simulink library "speedgoatlib_evse"  (R2024b)
settings: Solver=VariableStepAuto  StartTime=0.0  StopTime=10.0  RelTol=1e-3
undefined symbols (not defined in the file): sg_ev_charging_read_m, sg_ev_charging_write_m, sg_ev_isolation_read_m, sg_ev_parameter_read_m, sg_ev_parameter_write_m, sg_ev_precharge_read_m, sg_ev_precharge_write_m, sg_ev_status_m, sg_ev_stop_read_m, sg_ev_stop_write_m, sg_ev_welding_read_m, sg_ev_welding_write_m, sg_evse_charging_read_m, sg_evse_charging_write_m, sg_evse_isolation_read_m, sg_evse_isolation_write_m, sg_evse_parameter_read_m, sg_evse_parameter_write_m, sg_evse_precharge_read_m, sg_evse_precharge_write_m, sg_evse_status_m, sg_evse_stop_read_m, sg_evse_stop_write_m, sg_evse_welding_read_m, sg_evse_welding_write_m
libraries: speedgoatlib_mqtt x199, simulink x39, $bdroot x24
(part 6 of 8)

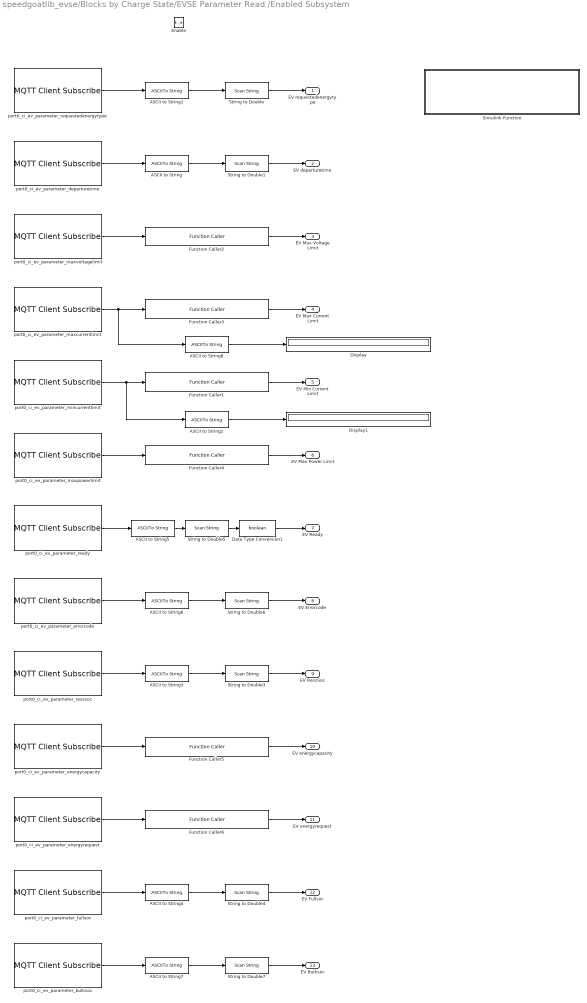
== system speedgoatlib_evse/Blocks by Charge State/EVSE Parameter Read /Enabled Subsystem ==
  Enable : EnablePort
  ASCII to String{,1..8} (9 alike) : ASCIIToString
  Data Type Conversion1 : DataTypeConversion  OutDataTypeStr=boolean  SaturateOnIntegerOverflow=off  RndMeth=Floor
  Display : Display
  Display1 : Display
  Function Caller{1..6} (6 alike) : FunctionCaller  FunctionPrototype=value = fromJsonPhysicalValue(uint8_vec)  InputArgumentSpecifications=zeros(1,48,'uint8')  OutputArgumentSpecifications=double(0)
  Simulink Function : Subsystem  TreatAsAtomicUnit=on
  String to Double{,1,3..7} (7 alike) : ScanString  Format="\"%lf\""
  port0_ci_ev_parameter_bulksoc : speedgoatlib_mqtt/Client/MQTT Client Subscribe  ClientId=parClientId  ConnectionId=parConnectionId  Topic='port0/ci/ev/parameter/bulksoc'  QoS=0 - at most once  InitValue=zeros(1,12,'uint8')  Extended=off  SampleTime=parSampleTime
      settings: SourceProductName=MQTT
  port0_ci_ev_parameter_departuretime : speedgoatlib_mqtt/Client/MQTT Client Subscribe  ClientId=parClientId  ConnectionId=parConnectionId  Topic='port0/ci/ev/parameter/departuretime'  QoS=0 - at most once  InitValue=zeros(1,24,'uint8')  Extended=off  SampleTime=parSampleTime
      settings: SourceProductName=MQTT
  port0_ci_ev_parameter_energycapacity : speedgoatlib_mqtt/Client/MQTT Client Subscribe  ClientId=parClientId  ConnectionId=parConnectionId  Topic='port0/ci/ev/parameter/energycapacity'  QoS=0 - at most once  InitValue=zeros(1,48,'uint8')  Extended=off  SampleTime=parSampleTime
      settings: SourceProductName=MQTT
  port0_ci_ev_parameter_energyrequest : speedgoatlib_mqtt/Client/MQTT Client Subscribe  ClientId=parClientId  ConnectionId=parConnectionId  Topic='port0/ci/ev/parameter/energyrequest'  QoS=0 - at most once  InitValue=zeros(1,48,'uint8')  Extended=off  SampleTime=parSampleTime
      settings: SourceProductName=MQTT
  port0_ci_ev_parameter_errorcode : speedgoatlib_mqtt/Client/MQTT Client Subscribe  ClientId=parClientId  ConnectionId=parConnectionId  Topic='port0/ci/ev/parameter/errorcode'  QoS=0 - at most once  InitValue=zeros(1,24,'uint8')  Extended=off  SampleTime=parSampleTime
      settings: SourceProductName=MQTT
  port0_ci_ev_parameter_fullsoc : speedgoatlib_mqtt/Client/MQTT Client Subscribe  ClientId=parClientId  ConnectionId=parConnectionId  Topic='port0/ci/ev/parameter/fullsoc'  QoS=0 - at most once  InitValue=zeros(1,12,'uint8')  Extended=off  SampleTime=parSampleTime
      settings: SourceProductName=MQTT
  port0_ci_ev_parameter_maxcurrentlimit : speedgoatlib_mqtt/Client/MQTT Client Subscribe  ClientId=parClientId  ConnectionId=parConnectionId  Topic='port0/ci/ev/parameter/maxcurrentlimit'  QoS=0 - at most once  InitValue=zeros(1,48,'uint8')  Extended=off  SampleTime=parSampleTime
      settings: SourceProductName=MQTT
  port0_ci_ev_parameter_maxpowerlimit : speedgoatlib_mqtt/Client/MQTT Client Subscribe  ClientId=parClientId  ConnectionId=parConnectionId  Topic='port0/ci/ev/parameter/maxpowerlimit'  QoS=0 - at most once  InitValue=zeros(1,48,'uint8')  Extended=off  SampleTime=parSampleTime
      settings: SourceProductName=MQTT
  port0_ci_ev_parameter_maxvoltagelimit : speedgoatlib_mqtt/Client/MQTT Client Subscribe  ClientId=parClientId  ConnectionId=parConnectionId  Topic='port0/ci/ev/parameter/maxvoltagelimit'  QoS=0 - at most once  InitValue=zeros(1,48,'uint8')  Extended=off  SampleTime=parSampleTime
      settings: SourceProductName=MQTT
  port0_ci_ev_parameter_mincurrentlimit : speedgoatlib_mqtt/Client/MQTT Client Subscribe  ClientId=parClientId  ConnectionId=parConnectionId  Topic='port0/ci/ev/parameter/mincurrentlimit'  QoS=0 - at most once  InitValue=zeros(1,48,'uint8')  Extended=off  SampleTime=parSampleTime
      settings: SourceProductName=MQTT
  port0_ci_ev_parameter_ready : speedgoatlib_mqtt/Client/MQTT Client Subscribe  ClientId=parClientId  ConnectionId=parConnectionId  Topic='port0/ci/ev/parameter/ready'  QoS=0 - at most once  InitValue=zeros(1,12,'uint8')  Extended=off  SampleTime=parSampleTime
      settings: SourceProductName=MQTT
  port0_ci_ev_parameter_requestedenergytype : speedgoatlib_mqtt/Client/MQTT Client Subscribe  ClientId=parClientId  ConnectionId=parConnectionId  Topic='port0/ci/ev/parameter/requestedenergytype'  QoS=0 - at most once  InitValue=zeros(1,12,'uint8')  Extended=off  SampleTime=parSampleTime
      settings: SourceProductName=MQTT
  port0_ci_ev_parameter_resssoc : speedgoatlib_mqtt/Client/MQTT Client Subscribe  ClientId=parClientId  ConnectionId=parConnectionId  Topic='port0/ci/ev/parameter/resssoc'  QoS=0 - at most once  InitValue=zeros(1,12,'uint8')  Extended=off  SampleTime=parSampleTime
      settings: SourceProductName=MQTT
  EV requestedenergytype : Outport
  EV departuretime : Outport  Port=2
  EV Max Voltage Limit : Outport  Port=3
  EV Max Current Limit : Outport  Port=4
  EV Min Current Limit : Outport  Port=5
  EV Max Power Limit : Outport  Port=6
  EV Ready : Outport  Port=7
  EV Errorcode : Outport  Port=8
  EV RessSoc : Outport  Port=9
  EV energycapacity : Outport  Port=10
  EV energyrequest : Outport  Port=11
  EV Fullsoc : Outport  Port=12
  EV Bulksoc : Outport  Port=13
  wires:
  String to Double/1 -> EV requestedenergytype/1
  port0_ci_ev_parameter_maxpowerlimit/1 -> Function Caller4/1
  Function Caller4/1 -> EV Max Power Limit/1
  Function Caller3/1 -> EV Max Current Limit/1
  port0_ci_ev_parameter_maxvoltagelimit/1 -> Function Caller2/1
  Function Caller2/1 -> EV Max Voltage Limit/1
  String to Double1/1 -> EV departuretime/1
  ASCII to String1/1 -> String to Double/1
  ASCII to String/1 -> String to Double1/1
  port0_ci_ev_parameter_departuretime/1 -> ASCII to String/1
  port0_ci_ev_parameter_requestedenergytype/1 -> ASCII to String1/1
  port0_ci_ev_parameter_mincurrentlimit/1 -> ASCII to String2/1, Function Caller1/1
  Function Caller1/1 -> EV Min Current Limit/1
  Data Type Conversion1/1 -> EV Ready/1
  String to Double5/1 -> Data Type Conversion1/1
  ASCII to String5/1 -> String to Double5/1
  port0_ci_ev_parameter_ready/1 -> ASCII to String5/1
  String to Double6/1 -> EV Errorcode/1
  ASCII to String6/1 -> String to Double6/1
  port0_ci_ev_parameter_errorcode/1 -> ASCII to String6/1
  port0_ci_ev_parameter_resssoc/1 -> ASCII to String3/1
  ASCII to String3/1 -> String to Double3/1
  String to Double3/1 -> EV RessSoc/1
  Function Caller5/1 -> EV energycapacity/1
  port0_ci_ev_parameter_energycapacity/1 -> Function Caller5/1
  port0_ci_ev_parameter_energyrequest/1 -> Function Caller6/1
  Function Caller6/1 -> EV energyrequest/1
  String to Double4/1 -> EV Fullsoc/1
  ASCII to String4/1 -> String to Double4/1
  port0_ci_ev_parameter_fullsoc/1 -> ASCII to String4/1
  port0_ci_ev_parameter_bulksoc/1 -> ASCII to String7/1
  ASCII to String7/1 -> String to Double7/1
  String to Double7/1 -> EV Bulksoc/1
  port0_ci_ev_parameter_maxcurrentlimit/1 -> ASCII to String8/1, Function Caller3/1
  ASCII to String8/1 -> Display/1
  ASCII to String2/1 -> Display1/1

== system speedgoatlib_evse/Blocks by Charge State/EVSE Parameter Read /string compare logic ==
  Input : Inport
  ASCII to String1 : ASCIIToString
  Add : Sum
  Data Type Conversion : DataTypeConversion  OutDataTypeStr=double  SaturateOnIntegerOverflow=off  RndMeth=Floor
  Data Type Conversion1 : DataTypeConversion  OutDataTypeStr=double  SaturateOnIntegerOverflow=off  RndMeth=Floor
  Gain : Gain  Gain=2
  String Compare : StringCompare
  String Compare1 : StringCompare
  String Constant : StringConstant  String="\"started\""
  String Constant1 : StringConstant  String="\"finished\""
  Out1 : Outport
  wires:
  ASCII to String1/1 -> String Compare1/1, String Compare/1
  String Constant1/1 -> String Compare1/2
  String Compare/1 -> Data Type Conversion/1
  String Constant/1 -> String Compare/2
  String Compare1/1 -> Data Type Conversion1/1
  Gain/1 -> Add/2
  Add/1 -> Out1/1
  Input/1 -> ASCII to String1/1
  Data Type Conversion/1 -> Add/1
  Data Type Conversion1/1 -> Gain/1

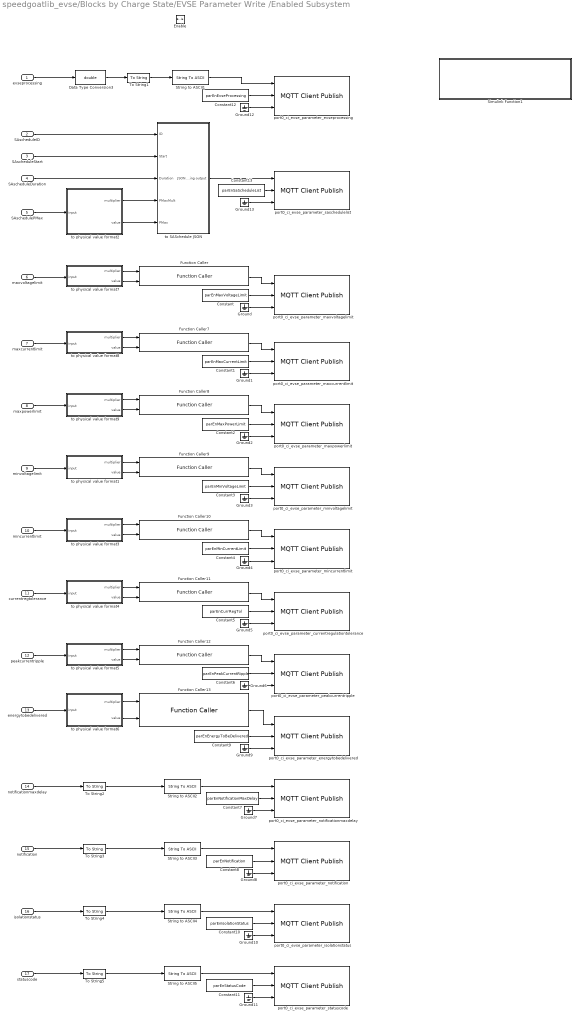
== system speedgoatlib_evse/Blocks by Charge State/EVSE Parameter Write /Enabled Subsystem ==
  evseprocessing : Inport
  SAscheduleID : Inport  Port=2
  SAscheduleStart : Inport  Port=3
  SAscheduleDuration : Inport  Port=4
  SAschedulePMax : Inport  Port=5
  maxvoltagelimit : Inport  Port=6
  maxcurrentlimit : Inport  Port=7
  maxpowerlimit : Inport  Port=8
  minvoltagelimit : Inport  Port=9
  mincurrentlimit : Inport  Port=10
  currentregtolerance : Inport  Port=11
  peakcurrentripple : Inport  Port=12
  energytobedelivered : Inport  Port=13
  notificationmaxdelay : Inport  Port=14
  notification : Inport  Port=15
  isolationstatus : Inport  Port=16
  statuscode : Inport  Port=17
  Enable : EnablePort
  Constant : Constant  Value=parEnMaxVoltageLimit  OutDataTypeStr=boolean
  Constant1 : Constant  Value=parEnMaxCurrentLimit  OutDataTypeStr=boolean
  Constant10 : Constant  Value=parEnIsolationStatus  OutDataTypeStr=boolean
  Constant11 : Constant  Value=parEnStatusCode  OutDataTypeStr=boolean
  Constant12 : Constant  Value=parEnEvseProcessing  OutDataTypeStr=boolean
  Constant13 : Constant  Value=parEnSaScheduleList  OutDataTypeStr=boolean
  Constant2 : Constant  Value=parEnMaxPowerLimit  OutDataTypeStr=boolean
  Constant3 : Constant  Value=parEnMinVoltageLimit  OutDataTypeStr=boolean
  Constant4 : Constant  Value=parEnMinCurrentLimit  OutDataTypeStr=boolean
  Constant5 : Constant  Value=parEnCurrRegTol  OutDataTypeStr=boolean
  Constant6 : Constant  Value=parEnPeakCurrentRipple  OutDataTypeStr=boolean
  Constant7 : Constant  Value=parEnNotificationMaxDelay  OutDataTypeStr=boolean
  Constant8 : Constant  Value=parEnNotification  OutDataTypeStr=boolean
  Constant9 : Constant  Value=parEnEnergyToBeDelivered  OutDataTypeStr=boolean
  Data Type Conversion3 : DataTypeConversion  OutDataTypeStr=double  SaturateOnIntegerOverflow=off  RndMeth=Floor
  Function Caller{,7..13} (8 alike) : FunctionCaller  FunctionPrototype=json_string = toJsonPhysicalValue(multiplier,value)  InputArgumentSpecifications=double(0), double(0)  OutputArgumentSpecifications=zeros(1,48,'uint8')
  Ground{,1..13} (14 alike) : Ground
  Simulink Function1 : Subsystem  TreatAsAtomicUnit=on
  String to ASCII1 : StringToASCII  OutputVectorSize=12
  String to ASCII2 : StringToASCII  OutputVectorSize=16
  String to ASCII3 : StringToASCII  OutputVectorSize=16
  String to ASCII4 : StringToASCII  OutputVectorSize=12
  String to ASCII5 : StringToASCII  OutputVectorSize=12
  To String{1..5} (5 alike) : ToString
  port0_ci_evse_parameter_currentregulationtolerance : speedgoatlib_mqtt/Client/MQTT Client Publish  ClientId=parClientId  ConnectionId=parConnectionId  Topic='port0/ci/evse/parameter/currentregulationtolerance'  QoS=0 - at most once  Retain=on  Extended=on  SampleTime=parSampleTime
      settings: SourceProductName=MQTT
  port0_ci_evse_parameter_energytobedelivered : speedgoatlib_mqtt/Client/MQTT Client Publish  ClientId=parClientId  ConnectionId=parConnectionId  Topic='port0/ci/evse/parameter/energytobedelivered'  QoS=0 - at most once  Retain=on  Extended=on  SampleTime=parSampleTime
      settings: SourceProductName=MQTT
  port0_ci_evse_parameter_evseprocessing : speedgoatlib_mqtt/Client/MQTT Client Publish  ClientId=parClientId  ConnectionId=parConnectionId  Topic='port0/ci/evse/parameter/evseprocessing'  QoS=0 - at most once  Retain=on  Extended=on  SampleTime=parSampleTime
      settings: SourceProductName=MQTT
  port0_ci_evse_parameter_isolationstatus : speedgoatlib_mqtt/Client/MQTT Client Publish  ClientId=parClientId  ConnectionId=parConnectionId  Topic='port0/ci/evse/parameter/isolationstatus'  QoS=0 - at most once  Retain=on  Extended=on  SampleTime=parSampleTime
      settings: SourceProductName=MQTT
  port0_ci_evse_parameter_maxcurrentlimit : speedgoatlib_mqtt/Client/MQTT Client Publish  ClientId=parClientId  ConnectionId=parConnectionId  Topic='port0/ci/evse/parameter/maxcurrentlimit'  QoS=0 - at most once  Retain=on  Extended=on  SampleTime=parSampleTime
      settings: SourceProductName=MQTT
  port0_ci_evse_parameter_maxpowerlimit : speedgoatlib_mqtt/Client/MQTT Client Publish  ClientId=parClientId  ConnectionId=parConnectionId  Topic='port0/ci/evse/parameter/maxpowerlimit'  QoS=0 - at most once  Retain=on  Extended=on  SampleTime=parSampleTime
      settings: SourceProductName=MQTT
  port0_ci_evse_parameter_maxvoltagelimit : speedgoatlib_mqtt/Client/MQTT Client Publish  ClientId=parClientId  ConnectionId=parConnectionId  Topic='port0/ci/evse/parameter/maxvoltagelimit'  QoS=0 - at most once  Retain=on  Extended=on  SampleTime=parSampleTime
      settings: SourceProductName=MQTT
  port0_ci_evse_parameter_mincurrentlimit : speedgoatlib_mqtt/Client/MQTT Client Publish  ClientId=parClientId  ConnectionId=parConnectionId  Topic='port0/ci/evse/parameter/mincurrentlimit'  QoS=0 - at most once  Retain=on  Extended=on  SampleTime=parSampleTime
      settings: SourceProductName=MQTT
  port0_ci_evse_parameter_minvoltagelimit : speedgoatlib_mqtt/Client/MQTT Client Publish  ClientId=parClientId  ConnectionId=parConnectionId  Topic='port0/ci/evse/parameter/minvoltagelimit'  QoS=0 - at most once  Retain=on  Extended=on  SampleTime=parSampleTime
      settings: SourceProductName=MQTT
  port0_ci_evse_parameter_notification : speedgoatlib_mqtt/Client/MQTT Client Publish  ClientId=parClientId  ConnectionId=parConnectionId  Topic='port0/ci/evse/parameter/notification'  QoS=0 - at most once  Retain=on  Extended=on  SampleTime=parSampleTime
      settings: SourceProductName=MQTT
  port0_ci_evse_parameter_notificationmaxdelay : speedgoatlib_mqtt/Client/MQTT Client Publish  ClientId=parClientId  ConnectionId=parConnectionId  Topic='port0/ci/evse/parameter/notificationmaxdelay'  QoS=0 - at most once  Retain=on  Extended=on  SampleTime=parSampleTime
      settings: SourceProductName=MQTT
  port0_ci_evse_parameter_peakcurrentripple : speedgoatlib_mqtt/Client/MQTT Client Publish  ClientId=parClientId  ConnectionId=parConnectionId  Topic='port0/ci/evse/parameter/peakcurrentripple'  QoS=0 - at most once  Retain=on  Extended=on  SampleTime=parSampleTime
      settings: SourceProductName=MQTT
  port0_ci_evse_parameter_saschedulelist : speedgoatlib_mqtt/Client/MQTT Client Publish  ClientId=parClientId  ConnectionId=parConnectionId  Topic='port0/ci/evse/parameter/saschedulelist'  QoS=0 - at most once  Retain=on  Extended=on  SampleTime=parSampleTime
      settings: SourceProductName=MQTT
  port0_ci_evse_parameter_statuscode : speedgoatlib_mqtt/Client/MQTT Client Publish  ClientId=parClientId  ConnectionId=parConnectionId  Topic='port0/ci/evse/parameter/statuscode'  QoS=0 - at most once  Retain=on  Extended=on  SampleTime=parSampleTime
      settings: SourceProductName=MQTT
  to SASchedule JSON : Subsystem
  to physical value format1 : MATLAB Function  TreatAsAtomicUnit=on
  to physical value format2 : MATLAB Function  TreatAsAtomicUnit=on
  to physical value format3 : MATLAB Function  TreatAsAtomicUnit=on
  to physical value format4 : MATLAB Function  TreatAsAtomicUnit=on
  to physical value format5 : MATLAB Function  TreatAsAtomicUnit=on
  to physical value format6 : MATLAB Function  TreatAsAtomicUnit=on
  to physical value format7 : MATLAB Function  TreatAsAtomicUnit=on
  to physical value format8 : MATLAB Function  TreatAsAtomicUnit=on
  to physical value format9 : MATLAB Function  TreatAsAtomicUnit=on
  wires:
  to physical value format6/2(value) -> Function Caller13/2
  to physical value format6/1(multiplier) -> Function Caller13/1
  Function Caller13/1 -> port0_ci_evse_parameter_energytobedelivered/1
  Function Caller12/1 -> port0_ci_evse_parameter_peakcurrentripple/1
  to physical value format5/2(value) -> Function Caller12/2
  to physical value format5/1(multiplier) -> Function Caller12/1
  Function Caller11/1 -> port0_ci_evse_parameter_currentregulationtolerance/1
  to physical value format4/2(value) -> Function Caller11/2
  to physical value format4/1(multiplier) -> Function Caller11/1
  Function Caller10/1 -> port0_ci_evse_parameter_mincurrentlimit/1
  to physical value format3/2(value) -> Function Caller10/2
  to physical value format3/1(multiplier) -> Function Caller10/1
  Function Caller9/1 -> port0_ci_evse_parameter_minvoltagelimit/1
  to physical value format1/2(value) -> Function Caller9/2
  to physical value format1/1(multiplier) -> Function Caller9/1
  Function Caller8/1 -> port0_ci_evse_parameter_maxpowerlimit/1
  to physical value format9/2(value) -> Function Caller8/2
  to physical value format9/1(multiplier) -> Function Caller8/1
  Function Caller7/1 -> port0_ci_evse_parameter_maxcurrentlimit/1
  to physical value format8/2(value) -> Function Caller7/2
  to physical value format8/1(multiplier) -> Function Caller7/1
  to physical value format7/2(value) -> Function Caller/2
  to physical value format7/1(multiplier) -> Function Caller/1
  Function Caller/1 -> port0_ci_evse_parameter_maxvoltagelimit/1
  Ground8/1 -> port0_ci_evse_parameter_notification/3
  Constant8/1 -> port0_ci_evse_parameter_notification/2
  Constant7/1 -> port0_ci_evse_parameter_notificationmaxdelay/2
  Ground7/1 -> port0_ci_evse_parameter_notificationmaxdelay/3
  Ground6/1 -> port0_ci_evse_parameter_peakcurrentripple/3
  Constant6/1 -> port0_ci_evse_parameter_peakcurrentripple/2
  Ground5/1 -> port0_ci_evse_parameter_currentregulationtolerance/3
  Constant5/1 -> port0_ci_evse_parameter_currentregulationtolerance/2
  Constant4/1 -> port0_ci_evse_parameter_mincurrentlimit/2
  Ground4/1 -> port0_ci_evse_parameter_mincurrentlimit/3
  Ground3/1 -> port0_ci_evse_parameter_minvoltagelimit/3
  Constant3/1 -> port0_ci_evse_parameter_minvoltagelimit/2
  Constant2/1 -> port0_ci_evse_parameter_maxpowerlimit/2
  Ground2/1 -> port0_ci_evse_parameter_maxpowerlimit/3
  Ground1/1 -> port0_ci_evse_parameter_maxcurrentlimit/3
  Constant1/1 -> port0_ci_evse_parameter_maxcurrentlimit/2
  Constant/1 -> port0_ci_evse_parameter_maxvoltagelimit/2
  Ground/1 -> port0_ci_evse_parameter_maxvoltagelimit/3
  evseprocessing/1 -> Data Type Conversion3/1
  statuscode/1 -> To String5/1
  String to ASCII5/1 -> port0_ci_evse_parameter_statuscode/1
  To String5/1 -> String to ASCII5/1
  To String4/1 -> String to ASCII4/1
  String to ASCII4/1 -> port0_ci_evse_parameter_isolationstatus/1
  isolationstatus/1 -> To String4/1
  notification/1 -> To String3/1
  String to ASCII3/1 -> port0_ci_evse_parameter_notification/1
  To String3/1 -> String to ASCII3/1
  To String2/1 -> String to ASCII2/1
  String to ASCII2/1 -> port0_ci_evse_parameter_notificationmaxdelay/1
  notificationmaxdelay/1 -> To String2/1
  energytobedelivered/1 -> to physical value format6/1(input)
  peakcurrentripple/1 -> to physical value format5/1(input)
  currentregtolerance/1 -> to physical value format4/1(input)
  minvoltagelimit/1 -> to physical value format1/1(input)
  mincurrentlimit/1 -> to physical value format3/1(input)
  to physical value format2/2(value) -> to SASchedule JSON/5(PMax)
  to physical value format2/1(multiplier) -> to SASchedule JSON/4(PMaxMult)
  SAscheduleDuration/1 -> to SASchedule JSON/3(Duration)
  SAscheduleStart/1 -> to SASchedule JSON/2(Start)
  SAscheduleID/1 -> to SASchedule JSON/1(ID)
  SAschedulePMax/1 -> to physical value format2/1(input)
  maxpowerlimit/1 -> to physical value format9/1(input)
  maxcurrentlimit/1 -> to physical value format8/1(input)
  maxvoltagelimit/1 -> to physical value format7/1(input)
  String to ASCII1/1 -> port0_ci_evse_parameter_evseprocessing/1
  to SASchedule JSON/1(JSON string output) -> port0_ci_evse_parameter_saschedulelist/1
  Data Type Conversion3/1 -> To String1/1
  To String1/1 -> String to ASCII1/1
  Constant9/1 -> port0_ci_evse_parameter_energytobedelivered/2
  Ground9/1 -> port0_ci_evse_parameter_energytobedelivered/3
  Constant10/1 -> port0_ci_evse_parameter_isolationstatus/2
  Ground10/1 -> port0_ci_evse_parameter_isolationstatus/3
  Ground11/1 -> port0_ci_evse_parameter_statuscode/3
  Constant11/1 -> port0_ci_evse_parameter_statuscode/2
  Ground12/1 -> port0_ci_evse_parameter_evseprocessing/3
  Constant12/1 -> port0_ci_evse_parameter_evseprocessing/2
  Constant13/1 -> port0_ci_evse_parameter_saschedulelist/2
  Ground13/1 -> port0_ci_evse_parameter_saschedulelist/3

== system speedgoatlib_evse/Blocks by Charge State/EVSE Parameter Write /string compare logic ==
  Input : Inport
  ASCII to String1 : ASCIIToString
  Add : Sum
  Data Type Conversion : DataTypeConversion  OutDataTypeStr=double  SaturateOnIntegerOverflow=off  RndMeth=Floor
  Data Type Conversion1 : DataTypeConversion  OutDataTypeStr=double  SaturateOnIntegerOverflow=off  RndMeth=Floor
  Gain : Gain  Gain=2
  String Compare : StringCompare
  String Compare1 : StringCompare
  String Constant : StringConstant  String="\"started\""
  String Constant1 : StringConstant  String="\"finished\""
  Out1 : Outport
  wires:
  Input/1 -> ASCII to String1/1
  Add/1 -> Out1/1
  Gain/1 -> Add/2
  String Compare1/1 -> Data Type Conversion1/1
  String Constant/1 -> String Compare/2
  String Compare/1 -> Data Type Conversion/1
  String Constant1/1 -> String Compare1/2
  ASCII to String1/1 -> String Compare/1, String Compare1/1
  Data Type Conversion/1 -> Add/1
  Data Type Conversion1/1 -> Gain/1

== system speedgoatlib_evse/Blocks by Charge State/EVSE Pre-Charge Read /Enabled Subsystem ==
  Enable : EnablePort
  ASCII to String : ASCIIToString
  ASCII to String1 : ASCIIToString
  ASCII to String2 : ASCIIToString
  Data Type Conversion1 : DataTypeConversion  OutDataTypeStr=boolean  SaturateOnIntegerOverflow=off  RndMeth=Floor
  Function Caller : FunctionCaller  FunctionPrototype=value = fromJsonPhysicalValue(uint8_vec)  InputArgumentSpecifications=zeros(1,48,'uint8')  OutputArgumentSpecifications=double(0)
  Function Caller1 : FunctionCaller  FunctionPrototype=value = fromJsonPhysicalValue(uint8_vec)  InputArgumentSpecifications=zeros(1,48,'uint8')  OutputArgumentSpecifications=double(0)
  Simulink Function : Subsystem  TreatAsAtomicUnit=on
  String to Double : ScanString  Format="\"%lf\""
  String to Double1 : ScanString  Format="\"%lf\""
  String to Double2 : ScanString  Format="\"%lf\""
  port0_ci_ev_precharge_errorcode : S-Function  FunctionName=sg_mqtt_client_subscribe_s  Parameters="ClientId,  ConnectionId, Topic, QoS, InitValue, Extended, SampleTime"  SFunctionDeploymentMode=off  EnableBusSupport=off  mask(mqtt_client_subscribe_1){ClientId=parClientId, ConnectionId=parConnectionId, Topic='port0/ci/ev/precharge/errorcode', QoS=0 - at most once, InitValue=zeros(1,24,'uint8'), Extended=off, SampleTime=parSampleTime}
      mask prompts: ClientId "Station ID"; ConnectionId "Connection ID"; QoS "Quality of Service"; InitValue "Init Value"; Extended "Extended Interface"; SampleTime "Sample Time [s]"
      mask help: Speedgoat Driver Block<br>MQTT Client - Subscribe<br><br>&copy; 2007 - 2023, Speedgoat GmbH, <a href="matlab: web('www.speedgoat.com','-browser');">www.speedgoat.com</a>
      mask init:
      | sg_mqtt_client_subscribe_m.runMaskInitialization(ClientId, ConnectionId, Topic, InitValue, Extended);
      mask Help: eval('sg.utils.help.show(''io_main/refentry_mqtt_client_subscribe'');')
      mask TypeOptions QoS: 0 - at most once | 1 - at least once | 2 - exactly once
      mask DialogControl groupParameters Prompt: Parameters
      mask Display: disp('Speedgoat\nMQTT Client\nSubscribe\nStation ID: 0\nConnection ID: 0');
  port0_ci_ev_precharge_ready : speedgoatlib_mqtt/Client/MQTT Client Subscribe  ClientId=parClientId  ConnectionId=parConnectionId  Topic='port0/ci/ev/precharge/ready'  QoS=0 - at most once  InitValue=zeros(1,12,'uint8')  Extended=off  SampleTime=parSampleTime
      settings: SourceProductName=MQTT
  port0_ci_ev_precharge_resssoc : S-Function  FunctionName=sg_mqtt_client_subscribe_s  Parameters="ClientId,  ConnectionId, Topic, QoS, InitValue, Extended, SampleTime"  SFunctionDeploymentMode=off  EnableBusSupport=off  mask(mqtt_client_subscribe_1){ClientId=parClientId, ConnectionId=parConnectionId, Topic='port0/ci/ev/precharge/resssoc', QoS=0 - at most once, InitValue=zeros(1,24,'uint8'), Extended=off, SampleTime=parSampleTime}
      mask prompts: ClientId "Station ID"; ConnectionId "Connection ID"; QoS "Quality of Service"; InitValue "Init Value"; Extended "Extended Interface"; SampleTime "Sample Time [s]"
      mask help: Speedgoat Driver Block<br>MQTT Client - Subscribe<br><br>&copy; 2007 - 2023, Speedgoat GmbH, <a href="matlab: web('www.speedgoat.com','-browser');">www.speedgoat.com</a>
      mask init:
      | sg_mqtt_client_subscribe_m.runMaskInitialization(ClientId, ConnectionId, Topic, InitValue, Extended);
      mask Help: eval('sg.utils.help.show(''io_main/refentry_mqtt_client_subscribe'');')
      mask TypeOptions QoS: 0 - at most once | 1 - at least once | 2 - exactly once
      mask DialogControl groupParameters Prompt: Parameters
      mask Display: disp('Speedgoat\nMQTT Client\nSubscribe\nStation ID: 0\nConnection ID: 0');
  port0_ci_ev_precharge_targetcurrent : S-Function  FunctionName=sg_mqtt_client_subscribe_s  Parameters="ClientId,  ConnectionId, Topic, QoS, InitValue, Extended, SampleTime"  SFunctionDeploymentMode=off  EnableBusSupport=off  mask(mqtt_client_subscribe_1){ClientId=parClientId, ConnectionId=parConnectionId, Topic='port0/ci/ev/precharge/targetcurrent', QoS=0 - at most once, InitValue=zeros(1,48,'uint8'), Extended=off, SampleTime=parSampleTime}
      mask prompts: ClientId "Station ID"; ConnectionId "Connection ID"; QoS "Quality of Service"; InitValue "Init Value"; Extended "Extended Interface"; SampleTime "Sample Time [s]"
      mask help: Speedgoat Driver Block<br>MQTT Client - Subscribe<br><br>&copy; 2007 - 2023, Speedgoat GmbH, <a href="matlab: web('www.speedgoat.com','-browser');">www.speedgoat.com</a>
      mask init:
      | sg_mqtt_client_subscribe_m.runMaskInitialization(ClientId, ConnectionId, Topic, InitValue, Extended);
      mask Help: eval('sg.utils.help.show(''io_main/refentry_mqtt_client_subscribe'');')
      mask TypeOptions QoS: 0 - at most once | 1 - at least once | 2 - exactly once
      mask DialogControl groupParameters Prompt: Parameters
      mask Display: disp('Speedgoat\nMQTT Client\nSubscribe\nStation ID: 0\nConnection ID: 0');
  port0_ci_ev_precharge_targetvoltage : S-Function  FunctionName=sg_mqtt_client_subscribe_s  Parameters="ClientId,  ConnectionId, Topic, QoS, InitValue, Extended, SampleTime"  SFunctionDeploymentMode=off  EnableBusSupport=off  mask(mqtt_client_subscribe_1){ClientId=parClientId, ConnectionId=parConnectionId, Topic='port0/ci/ev/precharge/targetvoltage', QoS=0 - at most once, InitValue=zeros(1,48,'uint8'), Extended=off, SampleTime=parSampleTime}
      mask prompts: ClientId "Station ID"; ConnectionId "Connection ID"; QoS "Quality of Service"; InitValue "Init Value"; Extended "Extended Interface"; SampleTime "Sample Time [s]"
      mask help: Speedgoat Driver Block<br>MQTT Client - Subscribe<br><br>&copy; 2007 - 2023, Speedgoat GmbH, <a href="matlab: web('www.speedgoat.com','-browser');">www.speedgoat.com</a>
      mask init:
      | sg_mqtt_client_subscribe_m.runMaskInitialization(ClientId, ConnectionId, Topic, InitValue, Extended);
      mask Help: eval('sg.utils.help.show(''io_main/refentry_mqtt_client_subscribe'');')
      mask TypeOptions QoS: 0 - at most once | 1 - at least once | 2 - exactly once
      mask DialogControl groupParameters Prompt: Parameters
      mask Display: disp('Speedgoat\nMQTT Client\nSubscribe\nStation ID: 0\nConnection ID: 0');
  EV Ready : Outport
  EV Errorcode : Outport  Port=2
  EV RESS SOC : Outport  Port=3
  EV Target Voltage : Outport  Port=4
  EV Target Current : Outport  Port=5
  wires:
  port0_ci_ev_precharge_ready/1 -> ASCII to String1/1
  port0_ci_ev_precharge_errorcode/1 -> ASCII to String/1
  ASCII to String/1 -> String to Double1/1
  ASCII to String1/1 -> String to Double/1
  String to Double/1 -> Data Type Conversion1/1
  String to Double1/1 -> EV Errorcode/1
  String to Double2/1 -> EV RESS SOC/1
  ASCII to String2/1 -> String to Double2/1
  port0_ci_ev_precharge_resssoc/1 -> ASCII to String2/1
  Function Caller/1 -> EV Target Voltage/1
  port0_ci_ev_precharge_targetvoltage/1 -> Function Caller/1
  port0_ci_ev_precharge_targetcurrent/1 -> Function Caller1/1
  Function Caller1/1 -> EV Target Current/1
  Data Type Conversion1/1 -> EV Ready/1

== system speedgoatlib_evse/Blocks by Charge State/EVSE Pre-Charge Read /string compare logic ==
  Input : Inport
  ASCII to String1 : ASCIIToString
  Add : Sum
  Gain : Gain  Gain=2
  String Compare : StringCompare
  String Compare1 : StringCompare
  String Constant : StringConstant  String="\"started\""
  String Constant1 : StringConstant  String="\"finished\""
  Out1 : Outport
  wires:
  Input/1 -> ASCII to String1/1
  Add/1 -> Out1/1
  Gain/1 -> Add/2
  String Compare1/1 -> Gain/1
  String Constant/1 -> String Compare/2
  String Compare/1 -> Add/1
  String Constant1/1 -> String Compare1/2
  ASCII to String1/1 -> String Compare/1, String Compare1/1

== system speedgoatlib_evse/Blocks by Charge State/EVSE Pre-Charge Write /Enabled Subsystem ==
  isolationstatus : Inport
  statuscode : Inport  Port=2
  presentvoltage : Inport  Port=3
  Enable : EnablePort
  Constant : Constant  Value=parEnIsolationStatus  OutDataTypeStr=boolean
  Constant1 : Constant  Value=parEnStatusCode  OutDataTypeStr=boolean
  Constant2 : Constant  Value=parEnPresentVoltage  OutDataTypeStr=boolean
  Data Type Conversion3 : DataTypeConversion  OutDataTypeStr=double  SaturateOnIntegerOverflow=off  RndMeth=Floor
  Data Type Conversion4 : DataTypeConversion  OutDataTypeStr=double  SaturateOnIntegerOverflow=off  RndMeth=Floor
  Function Caller11 : FunctionCaller  FunctionPrototype=json_string = toJsonPhysicalValue(multiplier,value)  InputArgumentSpecifications=double(0), double(0)  OutputArgumentSpecifications=zeros(1,48,'uint8')
  Ground : Ground
  Ground1 : Ground
  Ground2 : Ground
  Simulink Function2 : Subsystem  TreatAsAtomicUnit=on
  String to ASCII1 : StringToASCII  OutputVectorSize=12
  String to ASCII2 : StringToASCII  OutputVectorSize=12
  To String1 : ToString
  To String2 : ToString
  port0_ci_evse_precharge_isolationstatus : speedgoatlib_mqtt/Client/MQTT Client Publish  ClientId=parClientId  ConnectionId=parConnectionId  Topic='port0/ci/evse/precharge/isolationstatus'  QoS=0 - at most once  Retain=on  Extended=on  SampleTime=parSampleTime
      settings: SourceProductName=MQTT
  port0_ci_evse_precharge_presentvoltage : speedgoatlib_mqtt/Client/MQTT Client Publish  ClientId=parClientId  ConnectionId=parConnectionId  Topic='port0/ci/evse/precharge/presentvoltage'  QoS=0 - at most once  Retain=on  Extended=on  SampleTime=parSampleTime
      settings: SourceProductName=MQTT
  port0_ci_evse_precharge_statuscode : speedgoatlib_mqtt/Client/MQTT Client Publish  ClientId=parClientId  ConnectionId=parConnectionId  Topic='port0/ci/evse/precharge/statuscode'  QoS=0 - at most once  Retain=on  Extended=on  SampleTime=parSampleTime
      settings: SourceProductName=MQTT
  to physical value format : MATLAB Function  TreatAsAtomicUnit=on
  wires:
  to physical value format/2(value) -> Function Caller11/2
  to physical value format/1(multiplier) -> Function Caller11/1
  Function Caller11/1 -> port0_ci_evse_precharge_presentvoltage/1
  Data Type Conversion4/1 -> To String2/1
  To String2/1 -> String to ASCII2/1
  To String1/1 -> String to ASCII1/1
  Data Type Conversion3/1 -> To String1/1
  String to ASCII1/1 -> port0_ci_evse_precharge_isolationstatus/1
  String to ASCII2/1 -> port0_ci_evse_precharge_statuscode/1
  presentvoltage/1 -> to physical value format/1(input)
  isolationstatus/1 -> Data Type Conversion3/1
  statuscode/1 -> Data Type Conversion4/1
  Ground/1 -> port0_ci_evse_precharge_isolationstatus/3
  Constant/1 -> port0_ci_evse_precharge_isolationstatus/2
  Constant1/1 -> port0_ci_evse_precharge_statuscode/2
  Ground1/1 -> port0_ci_evse_precharge_statuscode/3
  Ground2/1 -> port0_ci_evse_precharge_presentvoltage/3
  Constant2/1 -> port0_ci_evse_precharge_presentvoltage/2

== system speedgoatlib_evse/Blocks by Charge State/EVSE Pre-Charge Write /string compare logic ==
  Input : Inport
  ASCII to String1 : ASCIIToString
  Add : Sum
  Gain : Gain  Gain=2
  String Compare : StringCompare
  String Compare1 : StringCompare
  String Constant : StringConstant  String="\"started\""
  String Constant1 : StringConstant  String="\"finished\""
  Out1 : Outport
  wires:
  ASCII to String1/1 -> String Compare1/1, String Compare/1
  String Constant1/1 -> String Compare1/2
  String Compare/1 -> Add/1
  String Constant/1 -> String Compare/2
  String Compare1/1 -> Gain/1
  Gain/1 -> Add/2
  Add/1 -> Out1/1
  Input/1 -> ASCII to String1/1

== system speedgoatlib_evse/Blocks by Charge State/EVSE Setup /Enabled Subsystem ==
  maxvoltagelimit : Inport
  maxcurrentlimit : Inport  Port=2
  mincurrentlimit : Inport  Port=3
  maxpowerlimit : Inport  Port=4
  minvoltagelimit : Inport  Port=5
  currentregtolerance : Inport  Port=6
  peakcurrentripple : Inport  Port=7
  Enable : EnablePort
  Function Caller{,1..6} (7 alike) : FunctionCaller  FunctionPrototype=json_string = toJsonPhysicalValue(multiplier,value)  InputArgumentSpecifications=double(0), double(0)  OutputArgumentSpecifications=zeros(1,48,'uint8')
  Function Caller7 : FunctionCaller  Commented=on  FunctionPrototype=json_string = toJsonPhysicalValue(multiplier,value)  InputArgumentSpecifications=double(0), double(0)  OutputArgumentSpecifications=zeros(1,48,'uint8')
  Simulink Function : Subsystem  TreatAsAtomicUnit=on
  port0_ci_evse_parameter_currentregulationtolerance : S-Function  FunctionName=sg_mqtt_client_publish_s  Parameters="ClientId,  ConnectionId, Topic, QoS, Retain, Extended, SampleTime"  SFunctionDeploymentMode=off  EnableBusSupport=off  mask(mqtt_client_publish_1){ClientId=parClientId, ConnectionId=parConnectionId, Topic='port0/ci/evse/parameter/currentregulationtolerance', QoS=0 - at most once, Retain=on, Extended=off, SampleTime=parSampleTime}
      mask prompts: ClientId "Station ID"; ConnectionId "Connection ID"; QoS "Quality of Service"; Extended "Extended Interface"; SampleTime "Sample Time [s]"
      mask help: Speedgoat Driver Block<br>MQTT Client - Publish<br><br>&copy; 2007 - 2023, Speedgoat GmbH, <a href="matlab: web('www.speedgoat.com','-browser');">www.speedgoat.com</a>
      mask init:
      | sg_mqtt_client_publish_m.runMaskInitialization(ClientId, ConnectionId, Topic, Extended);
      mask Help: eval('sg.utils.help.show(''io_main/refentry_mqtt_client_publish'');')
      mask TypeOptions QoS: 0 - at most once | 1 - at least once | 2 - exactly once
      mask DialogControl groupParameters Prompt: Parameters
      mask Display: disp('Speedgoat\nMQTT Client\nPublish\nStation ID: 0\nConnection ID: 0');
  port0_ci_evse_parameter_energytobedelivered : S-Function  Commented=on  FunctionName=sg_mqtt_client_publish_s  Parameters="ClientId,  ConnectionId, Topic, QoS, Retain, Extended, SampleTime"  SFunctionDeploymentMode=off  EnableBusSupport=off  mask(mqtt_client_publish_1){ClientId=parClientId, ConnectionId=parConnectionId, Topic='port0/ci/evse/parameter/energytobedelivered', QoS=0 - at most once, Retain=on, Extended=off, SampleTime=parSampleTime}
      mask prompts: ClientId "Station ID"; ConnectionId "Connection ID"; QoS "Quality of Service"; Extended "Extended Interface"; SampleTime "Sample Time [s]"
      mask help: Speedgoat Driver Block<br>MQTT Client - Publish<br><br>&copy; 2007 - 2023, Speedgoat GmbH, <a href="matlab: web('www.speedgoat.com','-browser');">www.speedgoat.com</a>
      mask init:
      | sg_mqtt_client_publish_m.runMaskInitialization(ClientId, ConnectionId, Topic, Extended);
      mask Help: eval('sg.utils.help.show(''io_main/refentry_mqtt_client_publish'');')
      mask TypeOptions QoS: 0 - at most once | 1 - at least once | 2 - exactly once
      mask DialogControl groupParameters Prompt: Parameters
      mask Display: disp('Speedgoat\nMQTT Client\nPublish\nStation ID: 0\nConnection ID: 0');
  port0_ci_evse_parameter_maxcurrentlimit : speedgoatlib_mqtt/Client/MQTT Client Publish  ClientId=parClientId  ConnectionId=parConnectionId  Topic='port0/ci/evse/parameter/maxcurrentlimit'  QoS=0 - at most once  Retain=on  Extended=off  SampleTime=parSampleTime
      settings: SourceProductName=MQTT
  port0_ci_evse_parameter_maxpowerlimit : speedgoatlib_mqtt/Client/MQTT Client Publish  ClientId=parClientId  ConnectionId=parConnectionId  Topic='port0/ci/evse/parameter/maxpowerlimit'  QoS=0 - at most once  Retain=on  Extended=off  SampleTime=parSampleTime
      settings: SourceProductName=MQTT
  port0_ci_evse_parameter_maxvoltagelimit : speedgoatlib_mqtt/Client/MQTT Client Publish  ClientId=parClientId  ConnectionId=parConnectionId  Topic='port0/ci/evse/parameter/maxvoltagelimit'  QoS=0 - at most once  Retain=on  Extended=off  SampleTime=parSampleTime
      settings: SourceProductName=MQTT
  port0_ci_evse_parameter_mincurrentlimit : speedgoatlib_mqtt/Client/MQTT Client Publish  ClientId=parClientId  ConnectionId=parConnectionId  Topic='port0/ci/evse/parameter/mincurrentlimit'  QoS=0 - at most once  Retain=on  Extended=off  SampleTime=parSampleTime
      settings: SourceProductName=MQTT
  port0_ci_evse_parameter_minvoltagelimit : S-Function  FunctionName=sg_mqtt_client_publish_s  Parameters="ClientId,  ConnectionId, Topic, QoS, Retain, Extended, SampleTime"  SFunctionDeploymentMode=off  EnableBusSupport=off  mask(mqtt_client_publish_1){ClientId=parClientId, ConnectionId=parConnectionId, Topic='port0/ci/evse/parameter/minvoltagelimit', QoS=0 - at most once, Retain=on, Extended=off, SampleTime=parSampleTime}
      mask prompts: ClientId "Station ID"; ConnectionId "Connection ID"; QoS "Quality of Service"; Extended "Extended Interface"; SampleTime "Sample Time [s]"
      mask help: Speedgoat Driver Block<br>MQTT Client - Publish<br><br>&copy; 2007 - 2023, Speedgoat GmbH, <a href="matlab: web('www.speedgoat.com','-browser');">www.speedgoat.com</a>
      mask init:
      | sg_mqtt_client_publish_m.runMaskInitialization(ClientId, ConnectionId, Topic, Extended);
      mask Help: eval('sg.utils.help.show(''io_main/refentry_mqtt_client_publish'');')
      mask TypeOptions QoS: 0 - at most once | 1 - at least once | 2 - exactly once
      mask DialogControl groupParameters Prompt: Parameters
      mask Display: disp('Speedgoat\nMQTT Client\nPublish\nStation ID: 0\nConnection ID: 0');
  port0_ci_evse_parameter_peakcurrentripple : S-Function  FunctionName=sg_mqtt_client_publish_s  Parameters="ClientId,  ConnectionId, Topic, QoS, Retain, Extended, SampleTime"  SFunctionDeploymentMode=off  EnableBusSupport=off  mask(mqtt_client_publish_1){ClientId=parClientId, ConnectionId=parConnectionId, Topic='port0/ci/evse/parameter/peakcurrentripple', QoS=0 - at most once, Retain=on, Extended=off, SampleTime=parSampleTime}
      mask prompts: ClientId "Station ID"; ConnectionId "Connection ID"; QoS "Quality of Service"; Extended "Extended Interface"; SampleTime "Sample Time [s]"
      mask help: Speedgoat Driver Block<br>MQTT Client - Publish<br><br>&copy; 2007 - 2023, Speedgoat GmbH, <a href="matlab: web('www.speedgoat.com','-browser');">www.speedgoat.com</a>
      mask init:
      | sg_mqtt_client_publish_m.runMaskInitialization(ClientId, ConnectionId, Topic, Extended);
      mask Help: eval('sg.utils.help.show(''io_main/refentry_mqtt_client_publish'');')
      mask TypeOptions QoS: 0 - at most once | 1 - at least once | 2 - exactly once
      mask DialogControl groupParameters Prompt: Parameters
      mask Display: disp('Speedgoat\nMQTT Client\nPublish\nStation ID: 0\nConnection ID: 0');
  to physical value format : MATLAB Function  TreatAsAtomicUnit=on
  to physical value format1 : MATLAB Function  TreatAsAtomicUnit=on
  to physical value format2 : MATLAB Function  TreatAsAtomicUnit=on
  to physical value format3 : MATLAB Function  TreatAsAtomicUnit=on
  to physical value format6 : MATLAB Function  TreatAsAtomicUnit=on
  to physical value format7 : MATLAB Function  TreatAsAtomicUnit=on
  to physical value format8 : MATLAB Function  TreatAsAtomicUnit=on
  to physical value format9 : MATLAB Function  Commented=on  TreatAsAtomicUnit=on
  wires:
  maxvoltagelimit/1 -> to physical value format/1(input)
  maxcurrentlimit/1 -> to physical value format1/1(input)
  mincurrentlimit/1 -> to physical value format2/1(input)
  maxpowerlimit/1 -> to physical value format3/1(input)
  minvoltagelimit/1 -> to physical value format6/1(input)
  currentregtolerance/1 -> to physical value format7/1(input)
  peakcurrentripple/1 -> to physical value format8/1(input)
  Function Caller/1 -> port0_ci_evse_parameter_maxvoltagelimit/1
  to physical value format/1(multiplier) -> Function Caller/1
  to physical value format/2(value) -> Function Caller/2
  to physical value format1/2(value) -> Function Caller1/2
  to physical value format1/1(multiplier) -> Function Caller1/1
  Function Caller1/1 -> port0_ci_evse_parameter_maxcurrentlimit/1
  Function Caller2/1 -> port0_ci_evse_parameter_mincurrentlimit/1
  to physical value format2/1(multiplier) -> Function Caller2/1
  to physical value format2/2(value) -> Function Caller2/2
  to physical value format3/2(value) -> Function Caller3/2
  to physical value format3/1(multiplier) -> Function Caller3/1
  Function Caller3/1 -> port0_ci_evse_parameter_maxpowerlimit/1
  Function Caller4/1 -> port0_ci_evse_parameter_minvoltagelimit/1
  to physical value format6/1(multiplier) -> Function Caller4/1
  to physical value format6/2(value) -> Function Caller4/2
  to physical value format7/2(value) -> Function Caller5/2
  to physical value format7/1(multiplier) -> Function Caller5/1
  Function Caller5/1 -> port0_ci_evse_parameter_currentregulationtolerance/1
  Function Caller6/1 -> port0_ci_evse_parameter_peakcurrentripple/1
  to physical value format8/1(multiplier) -> Function Caller6/1
  to physical value format8/2(value) -> Function Caller6/2
  to physical value format9/2(value) -> Function Caller7/2
  to physical value format9/1(multiplier) -> Function Caller7/1
  Function Caller7/1 -> port0_ci_evse_parameter_energytobedelivered/1

== system speedgoatlib_evse/Blocks by Charge State/EVSE Setup /string compare logic ==
  Input : Inport
  ASCII to String1 : ASCIIToString
  Add : Sum
  Data Type Conversion : DataTypeConversion  OutDataTypeStr=double  SaturateOnIntegerOverflow=off  RndMeth=Floor
  Data Type Conversion1 : DataTypeConversion  OutDataTypeStr=double  SaturateOnIntegerOverflow=off  RndMeth=Floor
  Gain : Gain  Gain=2
  String Compare : StringCompare
  String Compare1 : StringCompare
  String Constant : StringConstant  String="\"started\""
  String Constant1 : StringConstant  String="\"finished\""
  Out1 : Outport
  wires:
  ASCII to String1/1 -> String Compare1/1, String Compare/1
  String Constant1/1 -> String Compare1/2
  String Compare/1 -> Data Type Conversion/1
  String Constant/1 -> String Compare/2
  String Compare1/1 -> Data Type Conversion1/1
  Gain/1 -> Add/2
  Add/1 -> Out1/1
  Input/1 -> ASCII to String1/1
  Data Type Conversion/1 -> Add/1
  Data Type Conversion1/1 -> Gain/1

== system speedgoatlib_evse/Blocks by Charge State/EVSE Stop Read /Enabled Subsystem ==
  Enable : EnablePort
  ASCII to String : ASCIIToString
  String to Double1 : ScanString  Format="\"%lf\""
  port0_ci_ev_stop_progress : speedgoatlib_mqtt/Client/MQTT Client Subscribe  ClientId=parClientId  ConnectionId=parConnectionId  Topic='port0/ci/ev/stop/progress'  QoS=0 - at most once  InitValue=zeros(1,12,'uint8')  Extended=off  SampleTime=parSampleTime
      settings: SourceProductName=MQTT
  EV Stop Progress : Outport
  wires:
  ASCII to String/1 -> String to Double1/1
  String to Double1/1 -> EV Stop Progress/1
  port0_ci_ev_stop_progress/1 -> ASCII to String/1

== system speedgoatlib_evse/Blocks by Charge State/EVSE Stop Read /string compare logic ==
  Input : Inport
  ASCII to String1 : ASCIIToString
  Add : Sum
  Gain : Gain  Gain=2
  String Compare : StringCompare
  String Compare1 : StringCompare
  String Constant : StringConstant  String="\"started\""
  String Constant1 : StringConstant  String="\"finished\""
  Out1 : Outport
  wires:
  Input/1 -> ASCII to String1/1
  Add/1 -> Out1/1
  Gain/1 -> Add/2
  String Compare1/1 -> Gain/1
  String Constant/1 -> String Compare/2
  String Compare/1 -> Add/1
  String Constant1/1 -> String Compare1/2
  ASCII to String1/1 -> String Compare/1, String Compare1/1

== system speedgoatlib_evse/Blocks by Charge State/EVSE Stop Write /Enabled Subsystem ==
  stopProgress : Inport
  evseProcessing : Inport  Port=2
  Enable : EnablePort
  Constant1 : Constant  Value=parEnEvseProcessing  OutDataTypeStr=boolean
  Constant8 : Constant  Value=parEnStopProgress  OutDataTypeStr=boolean
  Data Type Conversion1 : DataTypeConversion  OutDataTypeStr=double  SaturateOnIntegerOverflow=off  RndMeth=Floor
  Data Type Conversion3 : DataTypeConversion  OutDataTypeStr=double  SaturateOnIntegerOverflow=off  RndMeth=Floor
  Ground1 : Ground
  Ground8 : Ground
  String to ASCII1 : StringToASCII  OutputVectorSize=12
  String to ASCII2 : StringToASCII  OutputVectorSize=12
  To String1 : ToString
  To String2 : ToString
  port0_ci_evse_stop_evseprocessing : speedgoatlib_mqtt/Client/MQTT Client Publish  ClientId=parClientId  ConnectionId=parConnectionId  Topic='port0/ci/evse/stop/evseprocessing'  QoS=0 - at most once  Retain=on  Extended=on  SampleTime=parSampleTime
      settings: SourceProductName=MQTT
  port0_ci_evse_stop_progress : speedgoatlib_mqtt/Client/MQTT Client Publish  ClientId=parClientId  ConnectionId=parConnectionId  Topic='port0/ci/evse/stop/progress'  QoS=0 - at most once  Retain=on  Extended=on  SampleTime=parSampleTime
      settings: SourceProductName=MQTT
  wires:
  evseProcessing/1 -> Data Type Conversion3/1
  Data Type Conversion3/1 -> To String1/1
  String to ASCII1/1 -> port0_ci_evse_stop_evseprocessing/1
  To String1/1 -> String to ASCII1/1
  Data Type Conversion1/1 -> To String2/1
  String to ASCII2/1 -> port0_ci_evse_stop_progress/1
  stopProgress/1 -> Data Type Conversion1/1
  To String2/1 -> String to ASCII2/1
  Ground8/1 -> port0_ci_evse_stop_progress/3
  Constant8/1 -> port0_ci_evse_stop_progress/2
  Constant1/1 -> port0_ci_evse_stop_evseprocessing/2
  Ground1/1 -> port0_ci_evse_stop_evseprocessing/3

== system speedgoatlib_evse/Blocks by Charge State/EVSE Stop Write /string compare logic ==
  Input : Inport
  ASCII to String1 : ASCIIToString
  Add : Sum
  Gain : Gain  Gain=2
  String Compare : StringCompare
  String Compare1 : StringCompare
  String Constant : StringConstant  String="\"started\""
  String Constant1 : StringConstant  String="\"finished\""
  Out1 : Outport
  wires:
  ASCII to String1/1 -> String Compare1/1, String Compare/1
  String Constant1/1 -> String Compare1/2
  String Compare/1 -> Add/1
  String Constant/1 -> String Compare/2
  String Compare1/1 -> Gain/1
  Gain/1 -> Add/2
  Add/1 -> Out1/1
  Input/1 -> ASCII to String1/1
